simulink model "Triggered2"  (R2020a)
settings: Solver=VariableStepAuto  StartTime=0.0  StopTime=5  RelTol=1e-3
settings Model: Creator=BEAR  LastModifiedBy=bzhan
settings DataIOCC: ReturnWorkspaceOutputs=off
settings DebuggingCC: ArithmeticOperatorsInVariantConditions=warning
settings SFSimCC: SimUseLocalCustomCode=off  CustomCodeUndefinedFunction=UseInterfaceOnly
settings RTWCC: RTWUseLocalCustomCode=off

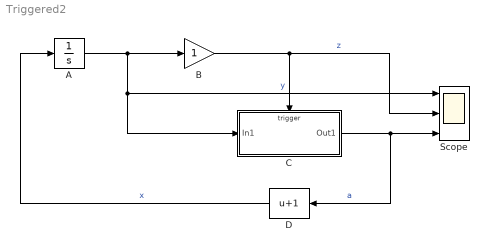
== system Triggered2 ==
  A : Integrator  InitialCondition=-1
  B : Gain  SampleTime=1
  C : Subsystem  TreatAsAtomicUnit=on
  D : Bias  Bias=1
  Scope : Scope  NumInputPorts=3
  wires:
  B/1 -> Scope/2, C/Trigger  "z"
  C/1(Out1) -> Scope/3, D/1  "a"
  D/1 -> A/1  "x"
  A/1 -> B/1, C/1(In1), Scope/1  "y"

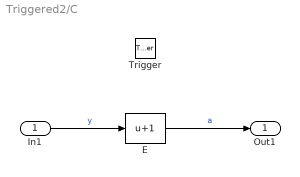
== system Triggered2/C ==
  In1 : Inport
  Trigger : TriggerPort  VariantControl=Variant
  E : Bias  Bias=1
  Out1 : Outport  VectorParamsAs1DForOutWhenUnconnected=off
  wires:
  E/1 -> Out1/1  "a"
  In1/1 -> E/1  "y"
